simulink model "LQR_pade_observer"  (R2023b)
settings: Solver=VariableStepAuto  StartTime=0.0  StopTime=100  RelTol=1e-3
values from neighbouring files (symbols this model uses):
  A = sys_pade.A    [attempt.m]    (also in model_approximation.m; observer.m = [-9.2083 0 8.1034; 1.0000 0 0; 0 0 -32.4138]; progetto.m = [0 1; 0 -1/Tm]; tuning.m)
  B = sys_pade.B    [attempt.m]    (also in model_approximation.m; observer.m = [-1;0;8]; progetto.m = [0 ;km/Tm]; tuning.m)
  C = sys_pade.C    [attempt.m]    (also in model_approximation.m; observer.m = [0, 6.486, 0]; progetto.m = [1 0]; tuning.m)
  D = sys_pade.D    [attempt.m]    (also in model_approximation.m; observer.m = 0; progetto.m = 0; tuning.m)
  K_tilde = [1.0710, 10.3987, 0.2638, -0.7581]    [observer.m]
  kr = -1/(C*inv(A-B*K_tilde(1:3))*B)    [controller_tuning.m]    (also in observer.m; progetto.m = -1/(C*inv(A-B*K)*B); tuning.m)
  L = eval(L)    [observer.m]    (also in torque.m = 0.0082)
  r = 50    [progetto.m]
undefined symbols (not defined in the file or in its folder): disturbance
settings Model: Creator=giova  LastModifiedBy=david

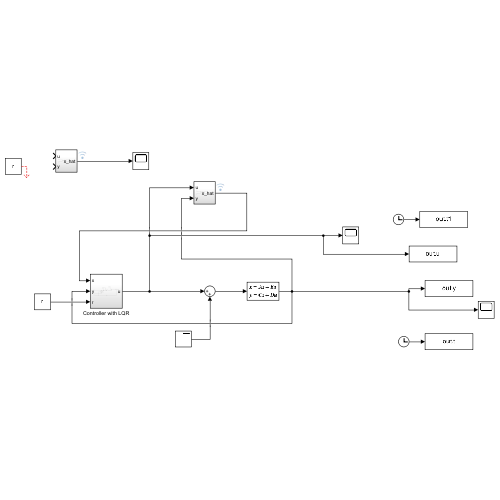
[thumbnail: Simulink's stored preview of the top-level diagram]
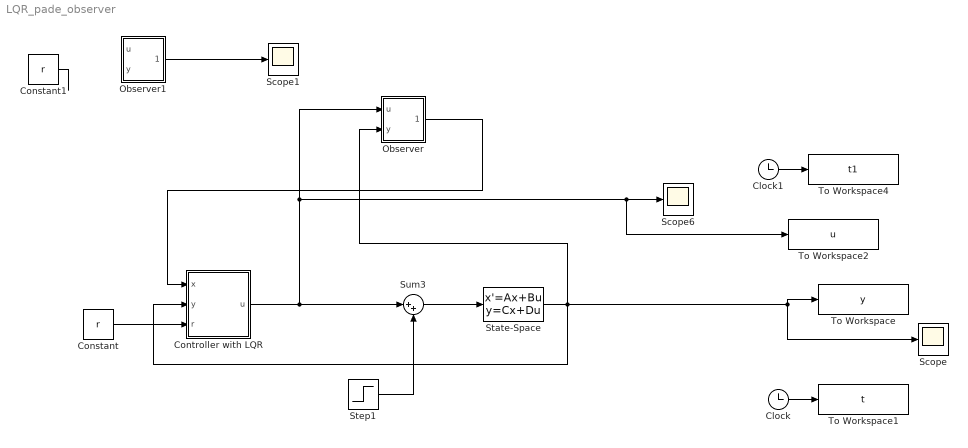
== system LQR_pade_observer ==
  Clock : Clock
  Clock1 : Clock
  Constant : Constant  Value=r
  Constant1 : Constant  Value=r
  Controller with LQR : Subsystem
  Observer : Subsystem
  Observer1 : Subsystem
  Scope : Scope
  Scope1 : Scope
  Scope6 : Scope
  State-Space : StateSpace  A=A  B=B  C=C  D=D  InitialCondition=0
  Step1 : Step  Time=2  After=disturbance  SampleTime=0
  Sum3 : Sum  Inputs=|++
  To Workspace : ToWorkspace  VariableName=y  SampleTime=-1
  To Workspace1 : ToWorkspace  VariableName=t  SampleTime=-1
  To Workspace2 : ToWorkspace  VariableName=u  SampleTime=-1
  To Workspace4 : ToWorkspace  VariableName=t1  SampleTime=-1
  wires:
  Sum3/1 -> State-Space/1
  Controller with LQR/1(u) -> To Workspace2/1, Scope6/1, Observer/1(u), Sum3/1
  Clock/1 -> To Workspace1/1
  Clock1/1 -> To Workspace4/1
  State-Space/1 -> To Workspace/1, Scope/1, Observer/2(y), Controller with LQR/2(y)
  Constant/1 -> Controller with LQR/3(r)
  Step1/1 -> Sum3/2
  Observer/1(x_hat) -> Controller with LQR/1(x)
  Constant1/1 -> ?
  Observer1/1(x_hat) -> Scope1/1

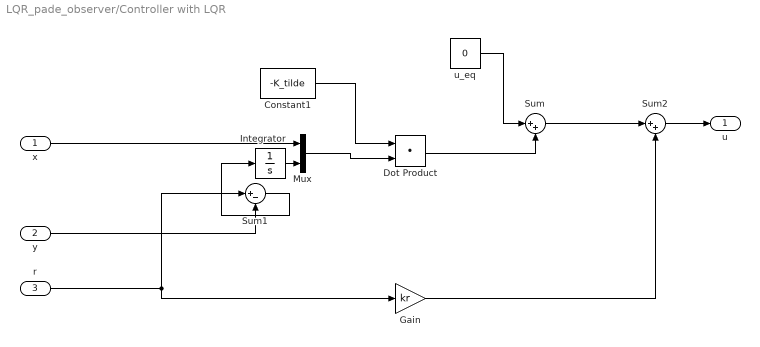
== system LQR_pade_observer/Controller with LQR ==
  x : Inport
  y : Inport  Port=2
  r : Inport  Port=3
  Constant1 : Constant  Value=-K_tilde
  Dot Product : DotProduct  OutDataTypeStr=Inherit: Inherit via internal rule
  Gain : Gain  Gain=kr
  Integrator : Integrator
  Mux : Mux  Inputs=2
  Sum : Sum  Inputs=|++
  Sum1 : Sum  Inputs=|+-
  Sum2 : Sum  Inputs=|++
  u_eq : Constant  Value=0
  u : Outport
  wires:
  r/1 -> Sum1/1, Gain/1
  Dot Product/1 -> Sum/2
  Sum/1 -> Sum2/1
  u_eq/1 -> Sum/1
  Gain/1 -> Sum2/2
  Constant1/1 -> Dot Product/1
  Sum2/1 -> u/1
  x/1 -> Mux/1
  Mux/1 -> Dot Product/2
  y/1 -> Sum1/2
  Integrator/1 -> Mux/2
  Sum1/1 -> Integrator/1

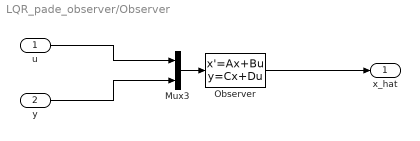
== system LQR_pade_observer/Observer ==
  u : Inport
  y : Inport  Port=2
  Mux3 : Mux  Inputs=2
  Observer : StateSpace  A=A-L*C  B=[B L]  C=eye(3)  D=[0 0; 0 0; 0 0]  InitialCondition=[0 0 0]  ParameterTunability=Unconstrained
  x_hat : Outport
  wires:
  y/1 -> Mux3/2
  u/1 -> Mux3/1
  Mux3/1 -> Observer/1
  Observer/1 -> x_hat/1

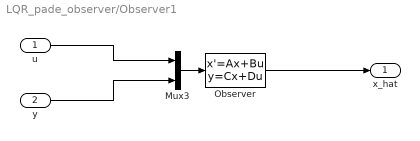
== system LQR_pade_observer/Observer1 ==
  u : Inport
  y : Inport  Port=2
  Mux3 : Mux  Inputs=2
  Observer : StateSpace  A=A-L*C  B=[B L]  C=eye(3)  D=[0 0; 0 0; 0 0]  InitialCondition=[0 r 0]  ParameterTunability=Unconstrained
  x_hat : Outport
  wires:
  y/1 -> Mux3/2
  u/1 -> Mux3/1
  Mux3/1 -> Observer/1
  Observer/1 -> x_hat/1
